simulink model "deimex"  (Simulink 8.5)
settings: Solver=ode45  SolverMode=SingleTasking  StartTime=0.0  StopTime=0.1  RelTol=1e-3  AbsTol=1e-6
libraries: elements x3, inputs x2
settings Model: Creator=PC  LastModifiedBy=PC
settings SolverCC: ZeroCrossAlgorithm=Adaptive
settings DataIOCC: LimitDataPoints=off
settings OptimizationCC: BlockReduction=off  BooleanDataType=off  ExpressionDepthLimit=128
settings DebuggingCC: SaveWithParameterizedLinksMsg=none  SignalResolutionControl=TryResolveAllWithWarning  MultiTaskDSMMsg=warning  MultiTaskCondExecSysMsg=none  FcnCallInpInsideContextMsg=EnableAllAsError  StateNameClashWarn=none
settings HardwareCC: TargetUnknown=on

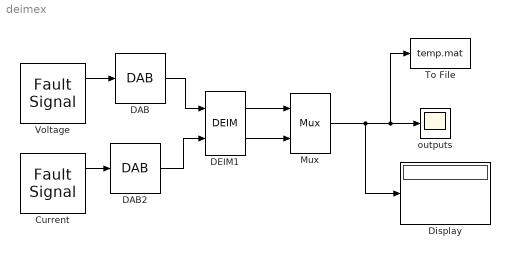
== system deimex ==
  Current : inputs/Fault Signal  pre_fault=[1 0]  post_fault=[10 90]  fr_dc=[60 2.25/60 0.0004]  oscA=[1.0 0.8 0.9]  oscf=[1000 3000 8000]  oscT=[0.050 0.030 0.060]
  DAB : elements/DAB  filter=on  approx=Bessel  order=2  numerator=[]  denominator=[]  freq=200  resdis=on  vertres=12  xmax=10  winsize=10  G=1.0  fs=60*20
  DAB2 : elements/DAB  filter=on  approx=Butterworth  order=2  numerator=[]  denominator=[]  freq=180  resdis=on  vertres=12  xmax=1  winsize=10  G=1.0  fs=60*20
  DEIM1 : elements/DEIM  type_pre=none  meth_sol=The least square method  num_meth=Euler  type_post=none  N=10  d=10  m=10  p=10  f=20*60  f1=60
  Display : Display
  Mux : Mux  Inputs=2
  To File : ToFile  Filename=temp.mat  MatrixName=y
  Voltage : inputs/Fault Signal  pre_fault=[10 0]  post_fault=[2 0]  fr_dc=[60 2.25/60 0.0004]  oscA=[1.0 0.8 0.9]  oscf=[1000 3000 8000]  oscT=[0.050 0.030 0.060]
  outputs : Scope
      settings: TickLabels=on  TimeRange=0.1  YMin=-2.25  YMax=0
  wires:
  Mux/1 -> Display/1, outputs/1, To File/1
  Voltage/1 -> DAB/1
  Current/1 -> DAB2/1
  DEIM1/2 -> Mux/2
  DEIM1/1 -> Mux/1
  DAB/1 -> DEIM1/1
  DAB2/1 -> DEIM1/2
